simulink model "H2DFRL_LExCI_env_TD3_nosfb"  (R2023a)
settings: Solver=FixedStepAuto  StartTime=0.0  StopTime=50  FixedStep=0.08  RelTol=1e-3
values from neighbouring files (symbols this model uses):
  action_mean_selector_ppo = 1:num_actions    [ReinforcementLearningBlockInit_H2DFRL.m]
  action_sampling_mode = 1    [ReinforcementLearningBlockInit_H2DFRL.m]
  action_selector_ddpg = 1:num_actions    [ReinforcementLearningBlockInit_H2DFRL.m]
  action_std_selector_ppo = 1:num_actions    [ReinforcementLearningBlockInit_H2DFRL.m]
  action_type = 1    [ReinforcementLearningBlockInit_H2DFRL.m]
  C2C_NMPC = init_C2C_NMPC_H2DF(C2C_NMPC.expdata)    [init_H2DFRL_GRU.m]
  LowerLimit = ([0.17e-3;350;-1;1.5e-3] - C2C_NMPC.Normalization.controls.mean)./(C2C_NMPC.Normalization.controls.std)    [init_H2DFRL_GRU.m]
  num_actions = 4    [ReinforcementLearningBlockInit_H2DFRL.m]
  rl_algorithm = 2    [ReinforcementLearningBlockInit_H2DFRL.m]
  Ts = 0.08    [init_H2DFRL_GRU.m]
  UpperLimit = ([0.5e-3;900;0;5.5e-3] - C2C_NMPC.Normalization.controls.mean)./(C2C_NMPC.Normalization.controls.std)    [init_H2DFRL_GRU.m]
undefined symbols (not defined in the file or in its folder): CA50_offset, DiscIntNeverNeededParam, enable_CA50_noise, enable_CA50_offset, enable_IMEP_noise, enable_IMEP_offset, IMEP_offset, NUMBER_OF_ACTIONS
libraries: simulink x15, dspsrcs4 x4, slctrlblks x2, statsLibrary x1
(part 1 of 4)
settings Model: Creator=sharma_v  LastModifiedBy=vasu3
settings DebuggingCC: ParameterPrecisionLossMsg=none

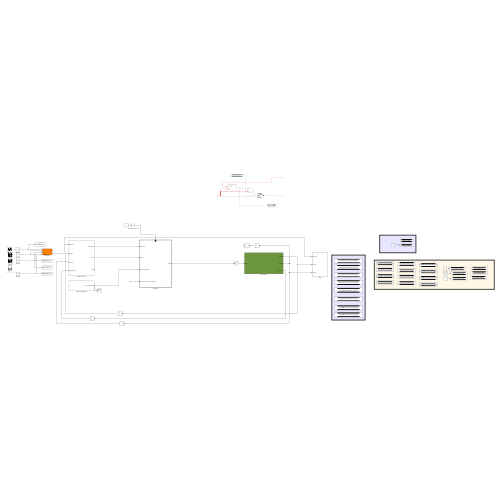
[thumbnail: Simulink's stored preview of the top-level diagram]
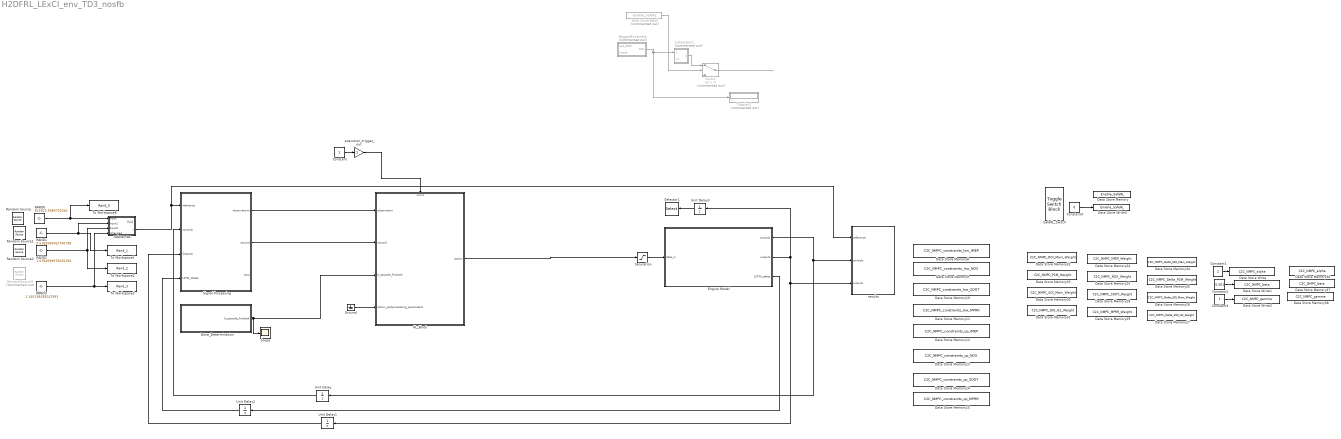
== system H2DFRL_LExCI_env_TD3_nosfb ==
  BaggedEnsemble : Subsystem  Commented=on
  Constant : Constant
  Constant1 : Constant  Value=2
  Constant2 : Constant  Value=0.001
  Constant3 : Constant
  Constant4 : Constant  Value=0
  Data Store Memory : DataStoreMemory  DataStoreName=Enable_SafeRL  WriteAfterWriteMsg=warning  ShowAdditionalParam=off
  Data Store Memory10 : DataStoreMemory  DataStoreName=C2C_NMPC_constraints_low_SOOT  WriteAfterWriteMsg=warning  ShowAdditionalParam=off
  Data Store Memory11 : DataStoreMemory  DataStoreName=C2C_NMPC_constraints_low_MPRR  WriteAfterWriteMsg=warning  ShowAdditionalParam=off
  Data Store Memory12 : DataStoreMemory  DataStoreName=C2C_NMPC_constraints_up_IMEP  WriteAfterWriteMsg=warning  ShowAdditionalParam=off
  Data Store Memory13 : DataStoreMemory  DataStoreName=C2C_NMPC_constraints_up_NOX  WriteAfterWriteMsg=warning  ShowAdditionalParam=off
  Data Store Memory14 : DataStoreMemory  DataStoreName=C2C_NMPC_constraints_up_SOOT  WriteAfterWriteMsg=warning  ShowAdditionalParam=off
  Data Store Memory15 : DataStoreMemory  DataStoreName=C2C_NMPC_constraints_up_MPRR  WriteAfterWriteMsg=warning  ShowAdditionalParam=off
  Data Store Memory24 : DataStoreMemory  DataStoreName=C2C_NMPC_IMEP_Weight  WriteAfterWriteMsg=warning  ShowAdditionalParam=off
  Data Store Memory25 : DataStoreMemory  DataStoreName=C2C_NMPC_NOX_Weight  WriteAfterWriteMsg=warning  ShowAdditionalParam=off
  Data Store Memory26 : DataStoreMemory  DataStoreName=C2C_NMPC_Delta_SOI_Main_Weight  WriteAfterWriteMsg=warning  ShowAdditionalParam=off
  Data Store Memory27 : DataStoreMemory  DataStoreName=C2C_NMPC_Delta_DOI_H2_Weight  WriteAfterWriteMsg=warning  ShowAdditionalParam=off
  Data Store Memory28 : DataStoreMemory  DataStoreName=C2C_NMPC_SOOT_Weight  WriteAfterWriteMsg=warning  ShowAdditionalParam=off
  Data Store Memory29 : DataStoreMemory  DataStoreName=C2C_NMPC_MPRR_Weight  WriteAfterWriteMsg=warning  ShowAdditionalParam=off
  Data Store Memory30 : DataStoreMemory  DataStoreName=C2C_NMPC_SOI_Main_Weight  WriteAfterWriteMsg=warning  ShowAdditionalParam=off
  Data Store Memory31 : DataStoreMemory  DataStoreName=C2C_NMPC_DOI_H2_Weight  WriteAfterWriteMsg=warning  ShowAdditionalParam=off
  Data Store Memory32 : DataStoreMemory  DataStoreName=C2C_NMPC_DOI_Main_Weight  WriteAfterWriteMsg=warning  ShowAdditionalParam=off
  Data Store Memory33 : DataStoreMemory  DataStoreName=C2C_NMPC_P2M_Weight  WriteAfterWriteMsg=warning  ShowAdditionalParam=off
  Data Store Memory34 : DataStoreMemory  DataStoreName=C2C_NMPC_Delta_DOI_Main_Weight  WriteAfterWriteMsg=warning  ShowAdditionalParam=off
  Data Store Memory35 : DataStoreMemory  DataStoreName=C2C_NMPC_Delta_P2M_Weight  WriteAfterWriteMsg=warning  ShowAdditionalParam=off
  Data Store Memory36 : DataStoreMemory  DataStoreName=C2C_NMPC_alpha  WriteAfterWriteMsg=warning  ShowAdditionalParam=off
  Data Store Memory37 : DataStoreMemory  DataStoreName=C2C_NMPC_beta  WriteAfterWriteMsg=warning  ShowAdditionalParam=off
  Data Store Memory38 : DataStoreMemory  DataStoreName=C2C_NMPC_gamma  WriteAfterWriteMsg=warning  ShowAdditionalParam=off
  Data Store Memory8 : DataStoreMemory  DataStoreName=C2C_NMPC_constraints_low_IMEP  WriteAfterWriteMsg=warning  ShowAdditionalParam=off
  Data Store Memory9 : DataStoreMemory  DataStoreName=C2C_NMPC_constraints_low_NOX  WriteAfterWriteMsg=warning  ShowAdditionalParam=off
  Data Store Read : DataStoreRead  Commented=on  DataStoreName=Enable_SafeRL  IndexOptions=Index vector (dialog)  Indices=1  OutputSizes=1
  Data Store Write : DataStoreWrite  DataStoreName=C2C_NMPC_alpha  IndexOptions=Index vector (dialog)  Indices=1  OutputSizes=1
  Data Store Write1 : DataStoreWrite  DataStoreName=C2C_NMPC_beta  IndexOptions=Index vector (dialog)  Indices=1  OutputSizes=1
  Data Store Write2 : DataStoreWrite  DataStoreName=C2C_NMPC_gamma  IndexOptions=Index vector (dialog)  Indices=1  OutputSizes=1
  Data Store Write3 : DataStoreWrite  DataStoreName=Enable_SafeRL  IndexOptions=Index vector (dialog)  Indices=1  OutputSizes=1
  Display2 : Display  Commented=on
  Done_Determination : Subsystem
  Engine Model : Subsystem
  Ground : Ground
  RAND0 : Constant  Value=815920.5980702044
  RAND1 : Constant  Value=0.5169590062740798
  RAND2 : Constant  Value=1.0784599976035294
  RAND3 : Constant  Value=1.140138438242993
  RL_Block : Subsystem
  Random Source : dspsrcs4/Random Source  SrcType=Uniform  NormMethod=Ziggurat  CltLength=12  MinVal=4e5  MaxVal=10e5  MeanVal=0  VarVal=1  RepMode=Not repeatable  rawSeed=1  IsInherit=off  SampMode=Discrete  SampTime=50  SampFrame=1  DataType=Double  OutComplex=Real  OutputFrames=off
  Random Source1 : dspsrcs4/Random Source  SrcType=Uniform  NormMethod=Ziggurat  CltLength=12  MinVal=0.5  MaxVal=1.3  MeanVal=0  VarVal=1  RepMode=Not repeatable  rawSeed=1  IsInherit=off  SampMode=Discrete  SampTime=50  SampFrame=1  DataType=Double  OutComplex=Real  OutputFrames=off
  Random Source2 : dspsrcs4/Random Source  SrcType=Uniform  NormMethod=Ziggurat  CltLength=12  MinVal=0.75  MaxVal=1.4  MeanVal=0  VarVal=1  RepMode=Not repeatable  rawSeed=1  IsInherit=off  SampMode=Discrete  SampTime=50  SampFrame=1  DataType=Double  OutComplex=Real  OutputFrames=off
  RandomSource3 : dspsrcs4/Random Source  Commented=on  SrcType=Uniform  NormMethod=Ziggurat  CltLength=12  MinVal=0.9  MaxVal=1.2  MeanVal=0  VarVal=1  RepMode=Not repeatable  rawSeed=1  IsInherit=off  SampMode=Discrete  SampTime=Tf  SampFrame=1  DataType=Double  OutComplex=Real  OutputFrames=off
  SafeRL_Switch : ToggleSwitchBlock
      settings: Values={{'Off', 'On'}, [0 1]}
  Saturation : Saturate  UpperLimit=[+1.4113;0.9867;0.9542; 2.1874]  LowerLimit=[-2.3201;-2.125;-1.8309; -1.6562]
  Scope : Scope
  Selector1 : Selector  IndexOptions=Index vector (dialog)  Indices=[1]  OutputSizes=1
  Signal Processing : Subsystem
  Subsystem1 : Subsystem  Commented=on
  Switch : Switch  Commented=on  Criteria=u2 > Threshold  SaturateOnIntegerOverflow=off  InputSameDT=off
  To Workspace1 : ToWorkspace  VariableName=Rand_1  SampleTime=-1
  To Workspace2 : ToWorkspace  VariableName=Rand_2  SampleTime=-1
  To Workspace3 : ToWorkspace  VariableName=Rand_3  SampleTime=-1
  To Workspace8 : ToWorkspace  VariableName=Rand_0  SampleTime=-1
  Unit Delay{,1..3} (4 alike) : UnitDelay  SampleTime=-1  HasFrameUpgradeWarning=on
  execution_trigger_out : Gain
  references : Subsystem
  results : Subsystem
  wires:
  RAND3/1 -> references/4(rchange4), To Workspace3/1
  Unit Delay1/1 -> Signal Processing/3(Outputs)
  RAND2/1 -> references/3(Input2), To Workspace2/1
  Unit Delay/1 -> Signal Processing/2(controls)
  RAND0/1 -> To Workspace8/1, references/1(Input)
  references/2(r) -> results/1(reference), Signal Processing/1(reference)
  RAND1/1 -> references/2(Input1), To Workspace1/1
  Unit Delay2/1 -> Signal Processing/4(LSTM_states)
  Constant2/1 -> Data Store Write1/1
  Engine Model/1(controls) -> Unit Delay/1, results/2(controls)
  Constant1/1 -> Data Store Write/1
  Constant3/1 -> Data Store Write2/1
  Engine Model/3(LSTM_states) -> Unit Delay2/1
  Signal Processing/1(observations) -> RL_Block/1(observation)
  Constant/1 -> execution_trigger_out/1
  Done_Determination/1(b_episode_finished) -> Scope/1, RL_Block/3(b_episode_finished)
  Ground/1 -> RL_Block/4(action_postprocessing_parameters)
  execution_trigger_out/1 -> RL_Block/Enable
  Signal Processing/2(reward) -> RL_Block/2(reward)
  Engine Model/2(outputs) -> Unit Delay1/1, results/3(outputs), Unit Delay3/1
  RL_Block/1("action ") -> Saturation/1
  Unit Delay3/1 -> Selector1/1
  Constant4/1 -> Data Store Write3/1
  Data Store Read/1 -> Switch/2
  BaggedEnsemble/1(NOx) -> Display2/1, Subsystem1/1(NOX)
  ? -> BaggedEnsemble/1(last_IMEP)
  Switch/1 -> ?
  ? -> BaggedEnsemble/2(Inputs), Subsystem1/2(u1), Switch/3
  Subsystem1/1(u*1) -> Switch/1
  Saturation/1 -> Engine Model/1(data_in)

== system H2DFRL_LExCI_env_TD3_nosfb/BaggedEnsemble ==
  last_IMEP : Inport
  Inputs : Inport  Port=2
  Mux : Mux  Inputs=2
  RegressionEnsemble Predict : statsLibrary/Regression/RegressionEnsemble Predict  TrainedLearner=trainedModel.RegressionEnsemble  OutMin=[]  OutMax=[]  WeakLearnerOutMin=[]  WeakLearnerOutMax=[]
  NOx : Outport
  wires:
  Mux/1 -> RegressionEnsemble Predict/1
  RegressionEnsemble Predict/1 -> NOx/1
  Inputs/1 -> Mux/1
  last_IMEP/1 -> Mux/2

== system H2DFRL_LExCI_env_TD3_nosfb/Done_Determination ==
  Clock : Clock  Commented=on
  Constant : Constant  Value=50
  Digital Clock : DigitalClock  SampleTime=-1
  Relational Operator : RelationalOperator  OutDataTypeStr=boolean  RndMeth=Simplest  InputSameDT=off
  b_episode_finished : Outport
  wires:
  Relational Operator/1 -> b_episode_finished/1
  Digital Clock/1 -> Relational Operator/1
  Constant/1 -> Relational Operator/2

== system H2DFRL_LExCI_env_TD3_nosfb/Engine Model ==
  data_in : Inport
  Delay1 : Delay  DelayLength=1  InitialCondition=C2C_NMPC.x0(1:C2C_NMPC.Dims.n_LSTM_states)
  Delay3 : Delay  DelayLength=1  InitialCondition=C2C_NMPC.x0
  Delay4 : Delay  DelayLength=1  InitialCondition=C2C_NMPC.x0((C2C_NMPC.Dims.n_states - C2C_NMPC.Dims.n_outputs + 1):C2C_NMPC.Dims.n_states)
  Mux2 : Mux  Inputs=2
  Mux3 : Mux  Inputs=2
  Selector1 : Selector  IndexOptions=Index vector (dialog)  Indices=[(C2C_NMPC.Dims.n_states - C2C_NMPC.Dims.n_outputs + 1):C2C_NMPC.Dims.n_states]  OutputSizes=1
  dyn_H2DF : Subsystem
  dyn_H2DF_state_augmentation : Subsystem
  offset_and_noise : Subsystem  Commented=on
  offset_and_noise1 : Subsystem
  controls : Outport
  outputs : Outport  Port=2
  LSTM_states : Outport  Port=3
  wires:
  Mux3/1 -> Delay3/1
  Delay1/1 -> dyn_H2DF/3(last_LSTM_states), dyn_H2DF_state_augmentation/1(last_LSTM_states)
  [controls] -> dyn_H2DF_state_augmentation/2(controls), Mux2/1
  Delay3/1 -> Selector1/1
  Delay4/1 -> dyn_H2DF_state_augmentation/3(last_outputs)
  Mux2/1 -> Mux3/2
  Selector1/1 -> dyn_H2DF/2(last_outputs)
  data_in/1 -> controls/1, [controls], dyn_H2DF/1(controls)
  dyn_H2DF/1(outputs) -> offset_and_noise1/1(outputs_in)
  dyn_H2DF_state_augmentation/1(LSTM_states) -> LSTM_states/1, Delay1/1, Mux3/1
  offset_and_noise1/1(outputs_out) -> Delay4/1, Mux2/2, outputs/1

== system H2DFRL_LExCI_env_TD3_nosfb/RL_Block ==
  observation : Inport
  reward : Inport  Port=2
  b_episode_finished : Inport  Port=3
  action_postprocessing_parameters : Inport  Port=4
  Enable : EnablePort
  Custom_Action_Postprocessing : Subsystem
  RL_Agent : Subsystem
  "action " : Outport
  wires:
  RL_Agent/1(action) -> Custom_Action_Postprocessing/1(rl_agent_action)
  action_postprocessing_parameters/1 -> Custom_Action_Postprocessing/2(action_postprocessing_parameters)
  b_episode_finished/1 -> RL_Agent/3(b_episode_finished)
  reward/1 -> RL_Agent/2(reward)
  observation/1 -> RL_Agent/1(observation)
  Custom_Action_Postprocessing/1("action ") -> "action "/1

== system H2DFRL_LExCI_env_TD3_nosfb/Signal Processing ==
  reference : Inport
  controls : Inport  Port=2
  Outputs : Inport  Port=3
  LSTM_states : Inport  Port=4
  Normalization : Subsystem  Commented=on
  calculate reward : Subsystem
  generate observations1 : Subsystem
  stop simulation : Subsystem
  observations : Outport
  reward : Outport  Port=2
  stop : Outport  Port=3
  wires:
  calculate reward/1(reward) -> reward/1
  stop simulation/1(stop) -> stop/1
  generate observations1/1(observations) -> observations/1
  reference/1 -> calculate reward/1(Reference), generate observations1/2(Reference)
  Outputs/1 -> stop simulation/1(Output), calculate reward/3(outputs), generate observations1/1(Outputs)
  controls/1 -> calculate reward/2(controls)
  LSTM_states/1 -> generate observations1/3(LSTM States)

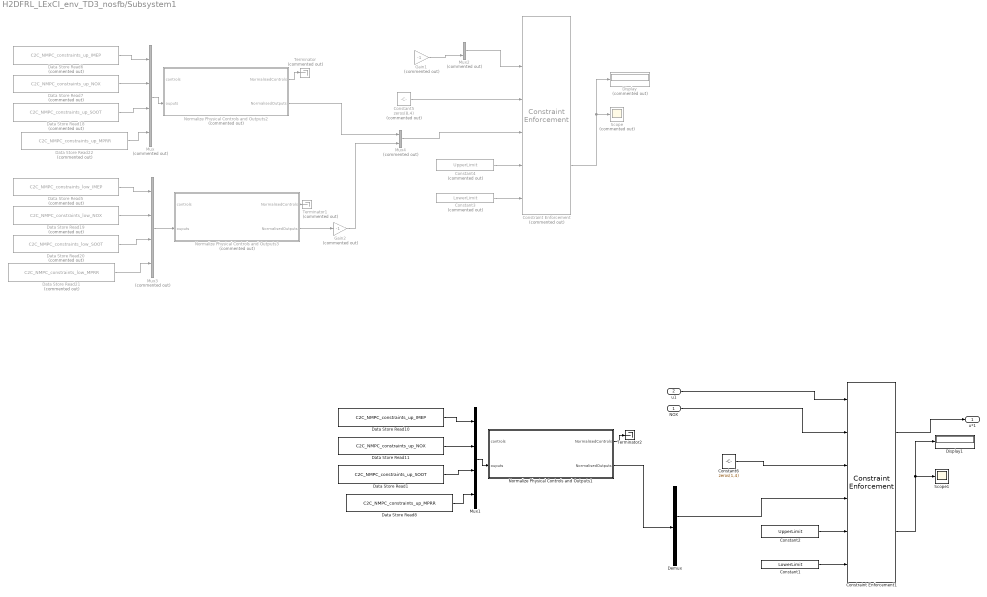
== system H2DFRL_LExCI_env_TD3_nosfb/Subsystem1 ==
  NOX : Inport
  u1 : Inport  Port=2
  Constant1 : Constant  Value=LowerLimit
  Constant2 : Constant  Value=UpperLimit
  Constant3 : Constant  Commented=on  Value=LowerLimit
  Constant4 : Constant  Commented=on  Value=UpperLimit
  Constant5 : Constant  Commented=on  Value=zeros(8,4)
  Constant6 : Constant  Value=zeros(1,4)
  Constraint Enforcement : slctrlblks/Constraint Enforcement  Commented=on  nc=8  nu=4  c=-0.14  external_c=on  external_umax=on  external_umin=on  Ts=0.08  maxiter=400  tol=1e-6  output_exitflag=on  relax_c=off  relax_u=off
  Constraint Enforcement1 : slctrlblks/Constraint Enforcement  nc=1  nu=4  c=-0.14  external_c=on  external_umax=on  external_umin=on  Ts=Ts  maxiter=400  tol=1e-3  output_exitflag=on  relax_c=off  relax_u=off
  Data Store Read1 : DataStoreRead  DataStoreName=C2C_NMPC_constraints_up_SOOT  IndexOptions=Index vector (dialog)  Indices=1  OutputSizes=1
  Data Store Read10 : DataStoreRead  DataStoreName=C2C_NMPC_constraints_up_IMEP  IndexOptions=Index vector (dialog)  Indices=1  OutputSizes=1
  Data Store Read11 : DataStoreRead  DataStoreName=C2C_NMPC_constraints_up_NOX  IndexOptions=Index vector (dialog)  Indices=1  OutputSizes=1
  Data Store Read18 : DataStoreRead  Commented=on  DataStoreName=C2C_NMPC_constraints_up_SOOT  IndexOptions=Index vector (dialog)  Indices=1  OutputSizes=1
  Data Store Read19 : DataStoreRead  Commented=on  DataStoreName=C2C_NMPC_constraints_low_NOX  IndexOptions=Index vector (dialog)  Indices=1  OutputSizes=1
  Data Store Read20 : DataStoreRead  Commented=on  DataStoreName=C2C_NMPC_constraints_low_SOOT  IndexOptions=Index vector (dialog)  Indices=1  OutputSizes=1
  Data Store Read21 : DataStoreRead  Commented=on  DataStoreName=C2C_NMPC_constraints_low_MPRR  IndexOptions=Index vector (dialog)  Indices=1  OutputSizes=1
  Data Store Read22 : DataStoreRead  Commented=on  DataStoreName=C2C_NMPC_constraints_up_MPRR  IndexOptions=Index vector (dialog)  Indices=1  OutputSizes=1
  Data Store Read5 : DataStoreRead  Commented=on  DataStoreName=C2C_NMPC_constraints_low_IMEP  IndexOptions=Index vector (dialog)  Indices=1  OutputSizes=1
  Data Store Read6 : DataStoreRead  Commented=on  DataStoreName=C2C_NMPC_constraints_up_IMEP  IndexOptions=Index vector (dialog)  Indices=1  OutputSizes=1
  Data Store Read7 : DataStoreRead  Commented=on  DataStoreName=C2C_NMPC_constraints_up_NOX  IndexOptions=Index vector (dialog)  Indices=1  OutputSizes=1
  Data Store Read8 : DataStoreRead  DataStoreName=C2C_NMPC_constraints_up_MPRR  IndexOptions=Index vector (dialog)  Indices=1  OutputSizes=1
  Demux : Demux
  Display : Display  Commented=on
  Display1 : Display
  Gain1 : Gain  Commented=on  Gain=-1
  Gain2 : Gain  Commented=on  Gain=-1
  Mux : Mux  Commented=on
  Mux1 : Mux
  Mux2 : Mux  Commented=on  Inputs=2
  Mux3 : Mux  Commented=on
  Mux4 : Mux  Commented=on  Inputs=2
  Normalize Physical Controls and Outputs1 : Subsystem
  Normalize Physical Controls and Outputs2 : Subsystem  Commented=on
  Normalize Physical Controls and Outputs3 : Subsystem  Commented=on
  Scope : Scope  Commented=on
  Scope1 : Scope
  Terminator : Terminator  Commented=on
  Terminator1 : Terminator  Commented=on
  Terminator2 : Terminator
  u*1 : Outport
  wires:
  Constant3/1 -> Constraint Enforcement/6
  Constant4/1 -> Constraint Enforcement/5
  Constant5/1 -> Constraint Enforcement/3
  Data Store Read18/1 -> Mux/3
  Data Store Read22/1 -> Mux/4
  Normalize Physical Controls and Outputs2/1("NormalisedControls ") -> Terminator/1
  Mux/1 -> Normalize Physical Controls and Outputs2/2("ouputs ")
  Data Store Read6/1 -> Mux/1
  Normalize Physical Controls and Outputs2/2(NormalisedOutputs) -> Mux4/1
  Data Store Read7/1 -> Mux/2
  Constraint Enforcement/2 -> Display/1, Scope/1
  Gain1/1 -> Mux2/2
  Mux2/1 -> Constraint Enforcement/2
  Data Store Read20/1 -> Mux3/3
  Normalize Physical Controls and Outputs3/1("NormalisedControls ") -> Terminator1/1
  Data Store Read21/1 -> Mux3/4
  Data Store Read19/1 -> Mux3/2
  Mux3/1 -> Normalize Physical Controls and Outputs3/2("ouputs ")
  Data Store Read5/1 -> Mux3/1
  Normalize Physical Controls and Outputs3/2(NormalisedOutputs) -> Gain2/1
  Gain2/1 -> Mux4/2
  Mux4/1 -> Constraint Enforcement/4
  Data Store Read10/1 -> Mux1/1
  Constraint Enforcement1/1 -> u*1/1
  Mux1/1 -> Normalize Physical Controls and Outputs1/2("ouputs ")
  Normalize Physical Controls and Outputs1/1("NormalisedControls ") -> Terminator2/1
  Data Store Read8/1 -> Mux1/4
  u1/1 -> Constraint Enforcement1/1
  Data Store Read1/1 -> Mux1/3
  NOX/1 -> Constraint Enforcement1/2
  Constant6/1 -> Constraint Enforcement1/3
  Constant1/1 -> Constraint Enforcement1/6
  Constant2/1 -> Constraint Enforcement1/5
  Data Store Read11/1 -> Mux1/2
  Normalize Physical Controls and Outputs1/2(NormalisedOutputs) -> Demux/1
  Demux/2 -> Constraint Enforcement1/4
  Constraint Enforcement1/2 -> Display1/1, Scope1/1

== system H2DFRL_LExCI_env_TD3_nosfb/references ==
  Input : Inport
  Input1 : Inport  Port=2
  Input2 : Inport  Port=3
  rchange4 : Inport  Port=4
  Clock : Clock
  Display : Display
  MATLAB Function : MATLAB Function  TreatAsAtomicUnit=on
  Mux : Mux  Inputs=2
  Mux1 : Mux  Inputs=2
  Mux2 : Mux
  Mux3 : Mux
  Normalize Reference Controls and Outputs : Subsystem
  Repeating Sequence Stair1 : simulink/Sources/Repeating Sequence Stair  OutValues=0  tsamp=-1  OutMin=[]  OutMax=[]  OutDataTypeStr=double  OutputDataTypeScalingMode=double  OutDataType=fixdt(0,8)  ConRadixGroup=Best Precision: Vector-wise  OutScaling=2^-12
  Reshape : Reshape  OutputDimensionality=Customize  OutputDimensions=[1,9]
  Subsystem1 : Subsystem
  Subsystem4 : Subsystem
  Out1 : Outport
  r : Outport  Port=2
  wires:
  Reshape/1 -> Out1/1
  Mux/1 -> Reshape/1
  Clock/1 -> MATLAB Function/1(t)
  Repeating Sequence Stair1/1 -> Mux/2
  Mux1/1 -> r/1, Display/1, Mux/1
  Input/1 -> MATLAB Function/2(rchange1)
  Input1/1 -> MATLAB Function/3(rchange2)
  Input2/1 -> MATLAB Function/4(rchange3)
  MATLAB Function/1(IMEP_ref) -> Mux2/1
  MATLAB Function/2(NOx_ref) -> Mux2/2
  MATLAB Function/3(SOOT_ref) -> Mux2/3
  MATLAB Function/4(MPRR_ref) -> Mux2/4
  Mux2/1 -> Normalize Reference Controls and Outputs/1("ouputs ")
  MATLAB Function/5(DOI_Main_ref) -> Mux3/1
  MATLAB Function/6(P2M_ref) -> Mux3/2
  MATLAB Function/7(SOI_ref) -> Mux3/3
  MATLAB Function/8(DOI_H2_ref) -> Mux3/4
  Mux3/1 -> Normalize Reference Controls and Outputs/2(controls)
  Normalize Reference Controls and Outputs/1(NormalisedOutputs) -> Mux1/1
  Normalize Reference Controls and Outputs/2("NormalisedControls ") -> Mux1/2
  rchange4/1 -> MATLAB Function/5(rchange4)

== system H2DFRL_LExCI_env_TD3_nosfb/results ==
  reference : Inport
  controls : Inport  Port=2
  outputs : Inport  Port=3
  Demux{1..4} (4 alike) : Demux
  Mux{1..3,7} (4 alike) : Mux  Inputs=2
  Mux6 : Mux
  Scope : Scope  NumInputPorts=8
  Scope2 : Scope
  Selector5 : Selector  IndexOptions=Index vector (dialog)  Indices=[1:4]  OutputSizes=1
  To Workspace : ToWorkspace  VariableName=IMEP  SampleTime=-1
  To Workspace1 : ToWorkspace  VariableName=NOX  SampleTime=-1
  To Workspace2 : ToWorkspace  VariableName=soot  SampleTime=-1
  To Workspace3 : ToWorkspace  VariableName=MPRR  SampleTime=-1
  To Workspace4 : ToWorkspace  VariableName=DOI_main  SampleTime=-1
  To Workspace5 : ToWorkspace  VariableName=SOI_pre  SampleTime=-1
  To Workspace6 : ToWorkspace  VariableName=SOI_main  SampleTime=-1
  To Workspace7 : ToWorkspace  VariableName=DOI_H2  SampleTime=-1
  To Workspace8 : ToWorkspace  VariableName=IMEP_RL  SampleTime=-1
  denormalizing physical controls and outputs : Subsystem
  denormalizing reference : Subsystem
  wires:
  reference/1 -> Selector5/1
  Selector5/1 -> Demux3/1
  outputs/1 -> Demux1/1
  controls/1 -> Demux2/1
  Mux7/1 -> To Workspace/1, Scope/1
  Mux2/1 -> To Workspace1/1, Scope/2
  Mux3/1 -> To Workspace3/1, Scope/4
  Mux1/1 -> To Workspace2/1, Scope/3
  Demux4/2 -> To Workspace5/1, Scope/6
  Demux4/3 -> To Workspace6/1, Scope/7
  Demux4/1 -> To Workspace4/1, Scope/5
  Mux6/1 -> Demux4/1
  Demux1/1 -> denormalizing physical controls and outputs/1(IMEP_norm)
  Demux1/2 -> denormalizing physical controls and outputs/2(NOX_norm)
  Demux1/3 -> denormalizing physical controls and outputs/3(soot_norm)
  Demux1/4 -> denormalizing physical controls and outputs/4(MPRR_norm)
  Demux2/1 -> denormalizing physical controls and outputs/5(DOI_main_norm)
  Demux2/2 -> denormalizing physical controls and outputs/6(SOI_pre_norm)
  Demux2/3 -> denormalizing physical controls and outputs/7(SOI_main_norm)
  denormalizing physical controls and outputs/1(IMEP) -> To Workspace8/1, Scope2/1, Mux7/2
  denormalizing physical controls and outputs/5(DOI_main) -> Mux6/1
  denormalizing physical controls and outputs/6(SOI_pre) -> Mux6/2
  denormalizing physical controls and outputs/7(SOI_main) -> Mux6/3
  denormalizing physical controls and outputs/2(NOX) -> Mux2/2
  denormalizing physical controls and outputs/3(soot) -> Mux1/2
  denormalizing physical controls and outputs/4(MPRR) -> Mux3/2
  Demux2/4 -> denormalizing physical controls and outputs/8(DOI_H2_norm)
  denormalizing physical controls and outputs/8(DOI_H2) -> Mux6/4
  Demux4/4 -> To Workspace7/1, Scope/8
  Demux3/1 -> denormalizing reference/1(IMEP_norm)
  Demux3/2 -> denormalizing reference/2(NOX_norm)
  Demux3/3 -> denormalizing reference/3(soot_norm)
  Demux3/4 -> denormalizing reference/4(MPRR_norm)
  denormalizing reference/1(IMEP) -> Mux7/1
  denormalizing reference/2(NOX) -> Mux2/1
  denormalizing reference/3(soot) -> Mux1/1
  denormalizing reference/4(MPRR) -> Mux3/1

== system H2DFRL_LExCI_env_TD3_nosfb/Engine Model/dyn_H2DF ==
  controls : Inport
  last_outputs : Inport  Port=2
  last_LSTM_states : Inport  Port=3
  dyn_H2DF : MATLAB Function  TreatAsAtomicUnit=on
  outputs : Outport
  LSTM_states : Outport  Port=2
  wires:
  dyn_H2DF/1(outputs) -> outputs/1
  controls/1 -> dyn_H2DF/2(controls)
  last_outputs/1 -> dyn_H2DF/3(last_outputs)
  dyn_H2DF/2(LSTM_states) -> LSTM_states/1
  last_LSTM_states/1 -> dyn_H2DF/1(last_LSTM_states)

== system H2DFRL_LExCI_env_TD3_nosfb/Engine Model/dyn_H2DF_state_augmentation ==
  last_LSTM_states : Inport
  controls : Inport  Port=2
  last_outputs : Inport  Port=3
  dyn_H2DF_state_augmentation : MATLAB Function  TreatAsAtomicUnit=on
  LSTM_states : Outport
  wires:
  dyn_H2DF_state_augmentation/1(LSTM_states) -> LSTM_states/1
  last_outputs/1 -> dyn_H2DF_state_augmentation/3(last_outputs)
  last_LSTM_states/1 -> dyn_H2DF_state_augmentation/1(last_LSTM_states)
  controls/1 -> dyn_H2DF_state_augmentation/2(controls)

== system H2DFRL_LExCI_env_TD3_nosfb/Engine Model/offset_and_noise ==
  outputs_in : Inport
  CA50_generation : Subsystem
  IMEP_generation : Subsystem
  Mux : Mux  Inputs=3
  Mux1 : Mux  Inputs=2
  Mux2 : Mux  Inputs=2
  Scope : Scope  NumInputPorts=2
  Selector1 : Selector  IndexOptions=Index vector (dialog)  Indices=[2, 3, 5]  OutputSizes=1
  Selector2 : Selector  IndexOptions=Index vector (dialog)  Indices=[4]  OutputSizes=1
  Selector3 : Selector  IndexOptions=Index vector (dialog)  Indices=[1]  OutputSizes=1
  outputs_out : Outport
  wires:
  Mux/1 -> outputs_out/1
  outputs_in/1 -> Selector3/1, Selector2/1, Selector1/1
  Selector3/1 -> Mux1/2, IMEP_generation/1(IMEP_in)
  Selector1/1 -> Mux/2
  IMEP_generation/1(IMEP_out) -> Mux1/1, Mux/1
  Selector2/1 -> CA50_generation/1(CA50_in), Mux2/2
  CA50_generation/1(CA50_out) -> Mux/3, Mux2/1
  Mux1/1 -> Scope/1
  Mux2/1 -> Scope/2

== system H2DFRL_LExCI_env_TD3_nosfb/Engine Model/offset_and_noise1 ==
  outputs_in : Inport
  IMEP_generation : Subsystem
  Mux : Mux  Inputs=2
  Mux1 : Mux  Inputs=2
  Scope : Scope  NumInputPorts=2
  Selector1 : Selector  IndexOptions=Index vector (dialog)  Indices=[2, 3, 4]  OutputSizes=1
  Selector3 : Selector  IndexOptions=Index vector (dialog)  Indices=[1]  OutputSizes=1
  outputs_out : Outport
  wires:
  Mux/1 -> outputs_out/1
  outputs_in/1 -> Selector3/1, Selector1/1
  Selector3/1 -> Mux1/2, Scope/2, IMEP_generation/1(IMEP_in)
  Selector1/1 -> Mux/2
  IMEP_generation/1(IMEP_out) -> Mux1/1, Mux/1
  Mux1/1 -> Scope/1

== system H2DFRL_LExCI_env_TD3_nosfb/RL_Block/Custom_Action_Postprocessing ==
  rl_agent_action : Inport
  action_postprocessing_parameters : Inport  Port=2
  Terminator : Terminator
  "action " : Outport
  wires:
  rl_agent_action/1 -> "action "/1
  action_postprocessing_parameters/1 -> Terminator/1
